simulink model "Casc_Filter_x4"  (Simulink 6.6)
settings: Solver=ode45  StartTime=0.0  StopTime=4100/sampling_freq  RelTol=1e-3
values from neighbouring files (symbols this model uses):
  filter_clk = sampling_freq*clk_mult    (= 144000000)    [Casecade_Taps.m]
  h_g = round(h_g*2^17)/2^17    [Casecade_Taps.m]
  h_k = round(h_k*2^17)/2^17    [Casecade_Taps.m]
  sampling_freq = 48e6    (= 48000000)    [Casecade_Taps.m]
undefined symbols (not defined in the file or in its folder): A, B, Fs, get, PCIN
libraries: xbsIndex_r4 x839, dspsnks4 x5, dspsrcs4 x1, simulink x1
(part 7 of 8)

== system Casc_Filter_x4/DDC/DDC C/Gaussian FIR Filters/Gaussian FIR Filter/Symmetric Data Flow ==
  Data In : Inport
  Counter : Inport  Port=2
  Counter Inv : Inport  Port=3
  Symmetric Shift Register : Subsystem
  Symmetric Shift Register1 : Subsystem
  Symmetric Shift Register2 : Subsystem
  Data 1 : Outport
  Data 2 : Outport  Port=2
  Data 3 : Outport  Port=3
  wires:
  Symmetric Shift Register/1(Shift Out 1) -> Symmetric Shift Register1/1(Shift In 1)
  Symmetric Shift Register1/3(Shift Out 2) -> Symmetric Shift Register/4(Shift In 2)
  Symmetric Shift Register/2(Sum Out) -> Data 1/1
  Symmetric Shift Register1/2(Sum Out) -> Data 2/1
  Data In/1 -> Symmetric Shift Register/1(Shift In 1)
  Counter/1 -> Symmetric Shift Register1/2(Counter), Symmetric Shift Register2/2(Counter), Symmetric Shift Register/2(Counter)
  Symmetric Shift Register1/1(Shift Out 1) -> Symmetric Shift Register2/1(Shift In 1)
  Symmetric Shift Register2/2(Sum Out) -> Data 3/1
  Symmetric Shift Register2/1(Shift Out 1) -> Symmetric Shift Register2/4(Shift In 2)
  Symmetric Shift Register2/3(Shift Out 2) -> Symmetric Shift Register1/4(Shift In 2)
  Counter Inv/1 -> Symmetric Shift Register/3(Counter Inv), Symmetric Shift Register1/3(Counter Inv), Symmetric Shift Register2/3(Counter Inv)

== system Casc_Filter_x4/DDC/DDC C/Gaussian FIR Filters/Gaussian FIR Filter1/Gaussian Accumulate ==
  Counter : Inport
  Data In : Inport  Port=2
  Constant : xbsIndex_r4/Constant  arith_type=Signed (2's comp)  const=0  n_bits=1  bin_pt=0  explicit_period=off  period=1  equ=P=C  opselect=C  inp2=PCIN>>17  opr=+  inp1=P  carry=CIN  dbl_ovrd=off  block_type=constant
      settings: block_version=VER_STRING_GOES_HERE
  Constant1 : xbsIndex_r4/Constant  arith_type=Signed (2's comp)  const=131071  n_bits=48  bin_pt=0  explicit_period=off  period=1  equ=P=P+1  opselect=Custom  inp2=P  opr=+  inp1=0  carry=1  dbl_ovrd=off  block_type=constant
      settings: block_version=VER_STRING_GOES_HERE
  Constant11 : xbsIndex_r4/Constant  arith_type=DSP48 Instruction  const=5  n_bits=7  bin_pt=0  explicit_period=off  period=1  equ=P=PCIN+(P)  opselect=Custom  inp2=PCIN  opr=+  inp1=P  carry=0  dbl_ovrd=off  block_type=constant
      settings: block_version=VER_STRING_GOES_HERE
  Constant2 : xbsIndex_r4/Constant  arith_type=Signed (2's comp)  const=0  n_bits=18  bin_pt=0  explicit_period=off  period=1  equ=P=P+1  opselect=Custom  inp2=P  opr=+  inp1=0  carry=1  dbl_ovrd=off  block_type=constant
      settings: block_version=VER_STRING_GOES_HERE
  Constant3 : xbsIndex_r4/Constant  arith_type=DSP48 Instruction  const=5  n_bits=7  bin_pt=0  explicit_period=off  period=1  equ=P=PCIN+(C)  opselect=Custom  inp2=PCIN  opr=+  inp1=C  carry=0  dbl_ovrd=off  block_type=constant
      settings: block_version=VER_STRING_GOES_HERE
  Constant6 : xbsIndex_r4/Constant  arith_type=Signed (2's comp)  const=0  n_bits=18  bin_pt=0  explicit_period=off  period=1  equ=P=P+1  opselect=Custom  inp2=P  opr=+  inp1=0  carry=1  dbl_ovrd=off  block_type=constant
      settings: block_version=VER_STRING_GOES_HERE
  DSP48 : xbsIndex_r4/DSP48  use_b=Direct from B Port  use_op=on  use_creg=on  use_pcin=on  use_pcout=off  use_bcout=off  rst_all=off  en_all=off  pipeline_a=0  pipeline_b=0  pipeline_c=off  pipeline_p=on  pipeline_mult=off  pipeline_opmode=on  pipeline_sub=off  pipeline_carryin=off  pipeline_carryinsel=off  rst_a=off  rst_b=off  rst_c=off  rst_mult=off  rst_p=off  rst_carry_in=off  rst_ctrl=off  en_a=off  en_b=off  en_c=off  en_mult=off  en_p=off  en_carry_in=off  en_ctrl=off  dbl_ovrd=off  use_synth_model=off  xl_useadderonly=on  block_type=dsp48
      settings: block_version=VER_STRING_GOES_HERE
  Delay1 : xbsIndex_r4/Delay  Orientation=down  en=off  latency=2  dbl_ovrd=off  reg_retiming=off  block_type=delay
      settings: infoedit=Hardware notes: A delay line is a chain, each link of which is an SRL16 followed by a flip-flop. If register retiming is enabled, the delay line is a chain of flip-flops.  block_version=VER_STRING_GOES_HERE
  Down Sample : xbsIndex_r4/Down Sample  sample_ratio=12  sample_phase="Last Value of Frame  (most efficient)"  en=off  latency=1  dbl_ovrd=off  block_type=dsamp
      settings: xl_area=[8 16 0 0 0 0 0]  block_version=VER_STRING_GOES_HERE
  Mux1 : xbsIndex_r4/Mux  inputs=2  en=off  latency=1  precision=Full  arith_type=Unsigned  n_bits=16  bin_pt=14  quantization=Truncate  overflow=Wrap  dbl_ovrd=off  block_type=mux
      settings: xl_area=[63 0 0 126 0 0 0]  block_version=VER_STRING_GOES_HERE
  Register : xbsIndex_r4/Register  Orientation=down  init=0  rst=off  en=on  dbl_ovrd=off  block_type=register
      settings: xl_area=[9 18 0 0 0 0 0]  block_version=VER_STRING_GOES_HERE
  Register1 : xbsIndex_r4/Register  init=0  rst=off  en=off  dbl_ovrd=off  block_type=register
      settings: block_version=8.2
  Reinterpret : xbsIndex_r4/Reinterpret  force_arith_type=on  arith_type="Signed  (2's comp)"  force_bin_pt=on  bin_pt=15  block_type=reinterpret
      settings: infoedit="Changes signal type without altering the binary representation.   You can changed the signal between signed and unsigned, and relocate the binary point.<P><P>Hardware notes: In hardware this block costs nothing.<P><P>Example:  Suppose the input is 6 bits wide, signed, with 2 fractional bits, and the output is forced to unsigned with 0 fractional bits.  Then an input of -2.0 (1110.00 in binary 2's complement) becomes an output of 56 (111000 in binary)."  block_version=8.2
  Relational : xbsIndex_r4/Relational  mode=a=b  en=off  latency=5  dbl_ovrd=off  block_type=relational
      settings: xl_area=[5 2 0 10 0 0 0]  block_version=VER_STRING_GOES_HERE
  Slice : xbsIndex_r4/Slice  nbits=16  boolean_output=off  mode=Lower Bit Location + Width  bit1=0  base1=MSB of Input  bit0=18  base0=LSB of Input  dbl_ovrd=off  block_type=slice
      settings: infoedit="Extracts a given range of bits from each input sample and presents it at the output.  The output type is ordinarily unsigned with binary point at zero, but can be Boolean when the slice is one bit wide.<P><P>Hardware notes: In hardware this block costs nothing."  block_version=VER_STRING_GOES_HERE
  Data Out : Outport
  wires:
  Constant/1 -> Relational/2
  Relational/1 -> Delay1/1, Mux1/1
  Counter/1 -> Relational/1
  Register/1 -> Down Sample/1
  Down Sample/1 -> Slice/1
  Delay1/1 -> Register/2
  Constant2/1 -> DSP48/1
  Constant6/1 -> DSP48/2
  Constant11/1 -> Mux1/2
  Constant3/1 -> Mux1/3
  DSP48/1 -> Register/1
  Slice/1 -> Reinterpret/1
  Register1/1 -> Data Out/1
  Mux1/1 -> DSP48/5
  Data In/1 -> DSP48/4
  Constant1/1 -> DSP48/3
  Reinterpret/1 -> Register1/1

== system Casc_Filter_x4/DDC/DDC C/Gaussian FIR Filters/Gaussian FIR Filter1/Gaussian Mult ==
  Data 1 : Inport
  Data 2 : Inport  Port=2
  Data 3 : Inport  Port=3
  Coeff 1 : Inport  Port=4
  Coeff 2 : Inport  Port=5
  Coeff 3 : Inport  Port=6
  Constant1 : xbsIndex_r4/Constant  arith_type=DSP48 Instruction  const=53  n_bits=7  bin_pt=0  explicit_period=off  period=1  equ=P=PCIN+(A*B)  opselect=PCIN + A*B  inp2=PCIN>>17  opr=+  inp1=P  carry=CIN  dbl_ovrd=off  block_type=constant
      settings: block_version=VER_STRING_GOES_HERE
  Constant2 : xbsIndex_r4/Constant  arith_type=DSP48 Instruction  const=53  n_bits=7  bin_pt=0  explicit_period=off  period=1  equ=P=PCIN+(A*B)  opselect=PCIN + A*B  inp2=PCIN>>17  opr=+  inp1=P  carry=CIN  dbl_ovrd=off  block_type=constant
      settings: block_version=VER_STRING_GOES_HERE
  Constant3 : xbsIndex_r4/Constant  arith_type=DSP48 Instruction  const=5  n_bits=7  bin_pt=0  explicit_period=off  period=1  equ=P=+(A*B)  opselect=A * B  inp2=PCIN>>17  opr=+  inp1=P  carry=CIN  dbl_ovrd=off  block_type=constant
      settings: block_version=VER_STRING_GOES_HERE
  DSP1 : xbsIndex_r4/DSP48  use_b=Direct from B Port  use_op=on  use_creg=off  use_pcin=on  use_pcout=on  use_bcout=off  rst_all=off  en_all=off  pipeline_a=2  pipeline_b=2  pipeline_c=on  pipeline_p=on  pipeline_mult=on  pipeline_opmode=off  pipeline_sub=off  pipeline_carryin=off  pipeline_carryinsel=off  rst_a=off  rst_b=off  rst_c=off  rst_mult=off  rst_p=off  rst_carry_in=off  rst_ctrl=off  en_a=off  en_b=off  en_c=off  en_mult=off  en_p=off  en_carry_in=off  en_ctrl=off  dbl_ovrd=off  use_synth_model=off  xl_useadderonly=off  block_type=dsp48
      settings: block_version=VER_STRING_GOES_HERE
  DSP3 : xbsIndex_r4/DSP48  use_b=Direct from B Port  use_op=on  use_creg=off  use_pcin=off  use_pcout=on  use_bcout=off  rst_all=off  en_all=off  pipeline_a=1  pipeline_b=1  pipeline_c=off  pipeline_p=on  pipeline_mult=on  pipeline_opmode=off  pipeline_sub=off  pipeline_carryin=off  pipeline_carryinsel=off  rst_a=off  rst_b=off  rst_c=off  rst_mult=off  rst_p=off  rst_carry_in=off  rst_ctrl=off  en_a=off  en_b=off  en_c=off  en_mult=off  en_p=off  en_carry_in=off  en_ctrl=off  dbl_ovrd=off  use_synth_model=off  xl_useadderonly=off  block_type=dsp48
      settings: block_version=VER_STRING_GOES_HERE
  DSP48 : xbsIndex_r4/DSP48  use_b=Direct from B Port  use_op=on  use_creg=off  use_pcin=on  use_pcout=on  use_bcout=off  rst_all=off  en_all=off  pipeline_a=2  pipeline_b=2  pipeline_c=on  pipeline_p=on  pipeline_mult=on  pipeline_opmode=off  pipeline_sub=off  pipeline_carryin=off  pipeline_carryinsel=off  rst_a=off  rst_b=off  rst_c=off  rst_mult=off  rst_p=off  rst_carry_in=off  rst_ctrl=off  en_a=off  en_b=off  en_c=off  en_mult=off  en_p=off  en_carry_in=off  en_ctrl=off  dbl_ovrd=off  use_synth_model=off  xl_useadderonly=off  block_type=dsp48
      settings: block_version=VER_STRING_GOES_HERE
  Delay1 : xbsIndex_r4/Delay  en=off  latency=2  dbl_ovrd=off  reg_retiming=off  block_type=delay
      settings: infoedit=Hardware notes: A delay line is a chain, each link of which is an SRL16 followed by a flip-flop. If register retiming is enabled, the delay line is a chain of flip-flops.  xl_area=[9 18 0 18 0 0 0]  block_version=VER_STRING_GOES_HERE
  Delay2 : xbsIndex_r4/Delay  en=off  latency=2  dbl_ovrd=off  reg_retiming=off  block_type=delay
      settings: infoedit=Hardware notes: A delay line is a chain, each link of which is an SRL16 followed by a flip-flop. If register retiming is enabled, the delay line is a chain of flip-flops.  xl_area=[9 18 0 18 0 0 0]  block_version=VER_STRING_GOES_HERE
  Delay3 : xbsIndex_r4/Delay  en=off  latency=3  dbl_ovrd=off  reg_retiming=off  block_type=delay
      settings: infoedit=Hardware notes: A delay line is a chain, each link of which is an SRL16 followed by a flip-flop. If register retiming is enabled, the delay line is a chain of flip-flops.  xl_area=[9 18 0 18 0 0 0]  block_version=VER_STRING_GOES_HERE
  Delay6 : xbsIndex_r4/Delay  en=off  latency=1  dbl_ovrd=off  reg_retiming=off  block_type=delay
      settings: infoedit=Hardware notes: A delay line is a chain, each link of which is an SRL16 followed by a flip-flop. If register retiming is enabled, the delay line is a chain of flip-flops.  xl_area=[9 18 0 18 0 0 0]  block_version=VER_STRING_GOES_HERE
  Reinterpret{,1..5} (6 alike) : xbsIndex_r4/Reinterpret  force_arith_type=on  arith_type="Signed  (2's comp)"  force_bin_pt=on  bin_pt=0  block_type=cast
      settings: infoedit="Changes type of samples without altering their binary representation.<P><P>Hardware notes: In hardware this block costs nothing.<P><P>Example:  Suppose the input is 6 bits wide, signed, with 2 fractional bits, and the output is forced to unsigned with 0 fractional bits.  Then an input of -2.0 (1110.00 in binary 2's complement) becomes an output of 56 (111000 in binary)."  block_version=VER_STRING_GOES_HERE
  Terminator : Terminator
  Terminator1 : Terminator
  Terminator2 : Terminator
  Sum Out : Outport
  wires:
  Data 1/1 -> Delay6/1
  Coeff 1/1 -> Delay3/1
  Data 3/1 -> Reinterpret/1
  Coeff 3/1 -> Delay1/1
  Delay1/1 -> Reinterpret1/1
  Delay3/1 -> Reinterpret5/1
  Delay6/1 -> Reinterpret4/1
  Coeff 2/1 -> Delay2/1
  Data 2/1 -> Reinterpret2/1
  Delay2/1 -> Reinterpret3/1
  Reinterpret/1 -> DSP3/1
  Reinterpret1/1 -> DSP3/2
  Constant3/1 -> DSP3/3
  DSP3/2 -> DSP48/3
  DSP3/1 -> Terminator/1
  Constant1/1 -> DSP48/4
  Reinterpret2/1 -> DSP48/1
  Reinterpret3/1 -> DSP48/2
  DSP48/2 -> DSP1/3
  DSP48/1 -> Terminator1/1
  Constant2/1 -> DSP1/4
  Reinterpret4/1 -> DSP1/1
  Reinterpret5/1 -> DSP1/2
  DSP1/1 -> Terminator2/1
  DSP1/2 -> Sum Out/1

== system Casc_Filter_x4/DDC/DDC C/Gaussian FIR Filters/Gaussian FIR Filter1/Symmetric Data Flow ==
  Data In : Inport
  Counter : Inport  Port=2
  Counter Inv : Inport  Port=3
  Symmetric Shift Register : Subsystem
  Symmetric Shift Register1 : Subsystem
  Symmetric Shift Register2 : Subsystem
  Data 1 : Outport
  Data 2 : Outport  Port=2
  Data 3 : Outport  Port=3
  wires:
  Symmetric Shift Register/1(Shift Out 1) -> Symmetric Shift Register1/1(Shift In 1)
  Symmetric Shift Register1/3(Shift Out 2) -> Symmetric Shift Register/4(Shift In 2)
  Symmetric Shift Register/2(Sum Out) -> Data 1/1
  Symmetric Shift Register1/2(Sum Out) -> Data 2/1
  Data In/1 -> Symmetric Shift Register/1(Shift In 1)
  Counter/1 -> Symmetric Shift Register1/2(Counter), Symmetric Shift Register2/2(Counter), Symmetric Shift Register/2(Counter)
  Symmetric Shift Register1/1(Shift Out 1) -> Symmetric Shift Register2/1(Shift In 1)
  Symmetric Shift Register2/2(Sum Out) -> Data 3/1
  Symmetric Shift Register2/1(Shift Out 1) -> Symmetric Shift Register2/4(Shift In 2)
  Symmetric Shift Register2/3(Shift Out 2) -> Symmetric Shift Register1/4(Shift In 2)
  Counter Inv/1 -> Symmetric Shift Register/3(Counter Inv), Symmetric Shift Register1/3(Counter Inv), Symmetric Shift Register2/3(Counter Inv)

== system Casc_Filter_x4/DDC/DDC A/Gaussian FIR Filters/Gaussian FIR Filter/Symmetric Data Flow/Symmetric Shift Register ==
  Shift In 1 : Inport
  Counter : Inport  Port=2
  Counter Inv : Inport  Port=3
  Shift In 2 : Inport  Port=4
  ASR : xbsIndex_r4/Addressable Shift Register  infer_latency=off  depth=12  initVector=[0]  en=off  dbl_ovrd=off  use_behavioral_HDL=off  use_rpm=off  block_type=addrsr
      settings: infoedit="Delay of  configurable length.  Any element  in the delay     line   can    be   addressed   and   driven    onto   the   output     port.<P><P>Hardware  notes: Implemented  using SRL16s.     If Virtex-4, Virtex-II or Spartan-3 devices are used, multiple SRLC16s are cascaded together."  xl_area=[9 0 0 18 0 0 0]  block_version=VER_STRING_GOES_HERE
  ASR1 : xbsIndex_r4/Addressable Shift Register  infer_latency=off  depth=12  initVector=[0]  en=off  dbl_ovrd=off  use_behavioral_HDL=off  use_rpm=off  block_type=addrsr
      settings: infoedit="Delay of  configurable length.  Any element  in the delay     line   can    be   addressed   and   driven    onto   the   output     port.<P><P>Hardware  notes: Implemented  using SRL16s.     If Virtex-4, Virtex-II or Spartan-3 devices are used, multiple SRLC16s are cascaded together."  xl_area=[9 0 0 18 0 0 0]  block_version=VER_STRING_GOES_HERE
  AddSub : xbsIndex_r4/AddSub  mode=Addition  use_carryin=off  use_carryout=off  en=off  latency=1  precision=User Defined  arith_type="Signed  (2's comp)"  n_bits=18  bin_pt=16  quantization="Round  (unbiased: +/- Inf)"  overflow=Saturate  dbl_ovrd=off  use_behavioral_HDL=off  pipelined=on  use_rpm=on  block_type=addsub
      settings: xl_area=[19 0 0 37 0 0 0]  block_version=VER_STRING_GOES_HERE
  Delay : xbsIndex_r4/Delay  en=off  latency=12  dbl_ovrd=off  reg_retiming=off  block_type=delay
      settings: infoedit=Hardware notes: A delay line is a chain, each link of which is an SRL16 followed by a flip-flop. If register retiming is enabled, the delay line is a chain of flip-flops.  xl_area=[9 18 0 18 0 0 0]  block_version=VER_STRING_GOES_HERE
  Delay1 : xbsIndex_r4/Delay  en=off  latency=12  dbl_ovrd=off  reg_retiming=off  block_type=delay
      settings: infoedit=Hardware notes: A delay line is a chain, each link of which is an SRL16 followed by a flip-flop. If register retiming is enabled, the delay line is a chain of flip-flops.  xl_area=[9 18 0 18 0 0 0]  block_version=VER_STRING_GOES_HERE
  Register : xbsIndex_r4/Register  init=0  rst=off  en=off  dbl_ovrd=off  block_type=register
      settings: block_version=8.2
  Register1 : xbsIndex_r4/Register  init=0  rst=off  en=off  dbl_ovrd=off  block_type=register
      settings: block_version=8.2
  Shift Out 1 : Outport
  Sum Out : Outport  Port=2
  Shift Out 2 : Outport  Port=3
  wires:
  Counter Inv/1 -> ASR1/2
  Shift In 1/1 -> ASR/1, Delay/1
  Shift In 2/1 -> Delay1/1, ASR1/1
  Counter/1 -> ASR/2
  ASR/1 -> Register/1
  ASR1/1 -> Register1/1
  AddSub/1 -> Sum Out/1
  Delay1/1 -> Shift Out 2/1
  Delay/1 -> Shift Out 1/1
  Register/1 -> AddSub/1
  Register1/1 -> AddSub/2

== system Casc_Filter_x4/DDC/DDC A/Gaussian FIR Filters/Gaussian FIR Filter/Symmetric Data Flow/Symmetric Shift Register1 ==
  Shift In 1 : Inport
  Counter : Inport  Port=2
  Counter Inv : Inport  Port=3
  Shift In 2 : Inport  Port=4
  ASR : xbsIndex_r4/Addressable Shift Register  infer_latency=off  depth=12  initVector=[0]  en=off  dbl_ovrd=off  use_behavioral_HDL=off  use_rpm=off  block_type=addrsr
      settings: infoedit="Delay of  configurable length.  Any element  in the delay     line   can    be   addressed   and   driven    onto   the   output     port.<P><P>Hardware  notes: Implemented  using SRL16s.     If Virtex-4, Virtex-II or Spartan-3 devices are used, multiple SRLC16s are cascaded together."  xl_area=[9 0 0 18 0 0 0]  block_version=VER_STRING_GOES_HERE
  ASR1 : xbsIndex_r4/Addressable Shift Register  infer_latency=off  depth=12  initVector=[0]  en=off  dbl_ovrd=off  use_behavioral_HDL=off  use_rpm=off  block_type=addrsr
      settings: infoedit="Delay of  configurable length.  Any element  in the delay     line   can    be   addressed   and   driven    onto   the   output     port.<P><P>Hardware  notes: Implemented  using SRL16s.     If Virtex-4, Virtex-II or Spartan-3 devices are used, multiple SRLC16s are cascaded together."  xl_area=[9 0 0 18 0 0 0]  block_version=VER_STRING_GOES_HERE
  AddSub : xbsIndex_r4/AddSub  mode=Addition  use_carryin=off  use_carryout=off  en=off  latency=1  precision=User Defined  arith_type="Signed  (2's comp)"  n_bits=18  bin_pt=16  quantization="Round  (unbiased: +/- Inf)"  overflow=Saturate  dbl_ovrd=off  use_behavioral_HDL=off  pipelined=on  use_rpm=on  block_type=addsub
      settings: xl_area=[19 0 0 37 0 0 0]  block_version=VER_STRING_GOES_HERE
  Delay : xbsIndex_r4/Delay  en=off  latency=12  dbl_ovrd=off  reg_retiming=off  block_type=delay
      settings: infoedit=Hardware notes: A delay line is a chain, each link of which is an SRL16 followed by a flip-flop. If register retiming is enabled, the delay line is a chain of flip-flops.  xl_area=[9 18 0 18 0 0 0]  block_version=VER_STRING_GOES_HERE
  Delay1 : xbsIndex_r4/Delay  en=off  latency=12  dbl_ovrd=off  reg_retiming=off  block_type=delay
      settings: infoedit=Hardware notes: A delay line is a chain, each link of which is an SRL16 followed by a flip-flop. If register retiming is enabled, the delay line is a chain of flip-flops.  xl_area=[9 18 0 18 0 0 0]  block_version=VER_STRING_GOES_HERE
  Register : xbsIndex_r4/Register  init=0  rst=off  en=off  dbl_ovrd=off  block_type=register
      settings: block_version=8.2
  Register1 : xbsIndex_r4/Register  init=0  rst=off  en=off  dbl_ovrd=off  block_type=register
      settings: block_version=8.2
  Shift Out 1 : Outport
  Sum Out : Outport  Port=2
  Shift Out 2 : Outport  Port=3
  wires:
  Counter Inv/1 -> ASR1/2
  Shift In 1/1 -> ASR/1, Delay/1
  Shift In 2/1 -> Delay1/1, ASR1/1
  Counter/1 -> ASR/2
  ASR/1 -> Register/1
  ASR1/1 -> Register1/1
  AddSub/1 -> Sum Out/1
  Delay1/1 -> Shift Out 2/1
  Delay/1 -> Shift Out 1/1
  Register/1 -> AddSub/1
  Register1/1 -> AddSub/2

== system Casc_Filter_x4/DDC/DDC A/Gaussian FIR Filters/Gaussian FIR Filter/Symmetric Data Flow/Symmetric Shift Register2 ==
  Shift In 1 : Inport
  Counter : Inport  Port=2
  Counter Inv : Inport  Port=3
  Shift In 2 : Inport  Port=4
  ASR : xbsIndex_r4/Addressable Shift Register  infer_latency=off  depth=12  initVector=[0]  en=off  dbl_ovrd=off  use_behavioral_HDL=off  use_rpm=off  block_type=addrsr
      settings: infoedit="Delay of  configurable length.  Any element  in the delay     line   can    be   addressed   and   driven    onto   the   output     port.<P><P>Hardware  notes: Implemented  using SRL16s.     If Virtex-4, Virtex-II or Spartan-3 devices are used, multiple SRLC16s are cascaded together."  xl_area=[9 0 0 18 0 0 0]  block_version=VER_STRING_GOES_HERE
  ASR1 : xbsIndex_r4/Addressable Shift Register  infer_latency=off  depth=12  initVector=[0]  en=off  dbl_ovrd=off  use_behavioral_HDL=off  use_rpm=off  block_type=addrsr
      settings: infoedit="Delay of  configurable length.  Any element  in the delay     line   can    be   addressed   and   driven    onto   the   output     port.<P><P>Hardware  notes: Implemented  using SRL16s.     If Virtex-4, Virtex-II or Spartan-3 devices are used, multiple SRLC16s are cascaded together."  xl_area=[9 0 0 18 0 0 0]  block_version=VER_STRING_GOES_HERE
  AddSub : xbsIndex_r4/AddSub  mode=Addition  use_carryin=off  use_carryout=off  en=off  latency=1  precision=User Defined  arith_type="Signed  (2's comp)"  n_bits=18  bin_pt=16  quantization="Round  (unbiased: +/- Inf)"  overflow=Saturate  dbl_ovrd=off  use_behavioral_HDL=off  pipelined=on  use_rpm=on  block_type=addsub
      settings: xl_area=[19 0 0 37 0 0 0]  block_version=VER_STRING_GOES_HERE
  Delay : xbsIndex_r4/Delay  en=off  latency=12  dbl_ovrd=off  reg_retiming=off  block_type=delay
      settings: infoedit=Hardware notes: A delay line is a chain, each link of which is an SRL16 followed by a flip-flop. If register retiming is enabled, the delay line is a chain of flip-flops.  xl_area=[9 18 0 18 0 0 0]  block_version=VER_STRING_GOES_HERE
  Delay1 : xbsIndex_r4/Delay  en=off  latency=12  dbl_ovrd=off  reg_retiming=off  block_type=delay
      settings: infoedit=Hardware notes: A delay line is a chain, each link of which is an SRL16 followed by a flip-flop. If register retiming is enabled, the delay line is a chain of flip-flops.  xl_area=[9 18 0 18 0 0 0]  block_version=VER_STRING_GOES_HERE
  Register : xbsIndex_r4/Register  init=0  rst=off  en=off  dbl_ovrd=off  block_type=register
      settings: block_version=8.2
  Register1 : xbsIndex_r4/Register  init=0  rst=off  en=off  dbl_ovrd=off  block_type=register
      settings: block_version=8.2
  Shift Out 1 : Outport
  Sum Out : Outport  Port=2
  Shift Out 2 : Outport  Port=3
  wires:
  Counter Inv/1 -> ASR1/2
  Shift In 1/1 -> ASR/1, Delay/1
  Shift In 2/1 -> Delay1/1, ASR1/1
  Counter/1 -> ASR/2
  ASR/1 -> Register/1
  ASR1/1 -> Register1/1
  AddSub/1 -> Sum Out/1
  Delay1/1 -> Shift Out 2/1
  Delay/1 -> Shift Out 1/1
  Register/1 -> AddSub/1
  Register1/1 -> AddSub/2

== system Casc_Filter_x4/DDC/DDC A/Gaussian FIR Filters/Gaussian FIR Filter1/Symmetric Data Flow/Symmetric Shift Register ==
  Shift In 1 : Inport
  Counter : Inport  Port=2
  Counter Inv : Inport  Port=3
  Shift In 2 : Inport  Port=4
  ASR : xbsIndex_r4/Addressable Shift Register  infer_latency=off  depth=12  initVector=[0]  en=off  dbl_ovrd=off  use_behavioral_HDL=off  use_rpm=off  block_type=addrsr
      settings: infoedit="Delay of  configurable length.  Any element  in the delay     line   can    be   addressed   and   driven    onto   the   output     port.<P><P>Hardware  notes: Implemented  using SRL16s.     If Virtex-4, Virtex-II or Spartan-3 devices are used, multiple SRLC16s are cascaded together."  xl_area=[9 0 0 18 0 0 0]  block_version=VER_STRING_GOES_HERE
  ASR1 : xbsIndex_r4/Addressable Shift Register  infer_latency=off  depth=12  initVector=[0]  en=off  dbl_ovrd=off  use_behavioral_HDL=off  use_rpm=off  block_type=addrsr
      settings: infoedit="Delay of  configurable length.  Any element  in the delay     line   can    be   addressed   and   driven    onto   the   output     port.<P><P>Hardware  notes: Implemented  using SRL16s.     If Virtex-4, Virtex-II or Spartan-3 devices are used, multiple SRLC16s are cascaded together."  xl_area=[9 0 0 18 0 0 0]  block_version=VER_STRING_GOES_HERE
  AddSub : xbsIndex_r4/AddSub  mode=Addition  use_carryin=off  use_carryout=off  en=off  latency=1  precision=User Defined  arith_type="Signed  (2's comp)"  n_bits=18  bin_pt=16  quantization="Round  (unbiased: +/- Inf)"  overflow=Saturate  dbl_ovrd=off  use_behavioral_HDL=off  pipelined=on  use_rpm=on  block_type=addsub
      settings: xl_area=[19 0 0 37 0 0 0]  block_version=VER_STRING_GOES_HERE
  Delay : xbsIndex_r4/Delay  en=off  latency=12  dbl_ovrd=off  reg_retiming=off  block_type=delay
      settings: infoedit=Hardware notes: A delay line is a chain, each link of which is an SRL16 followed by a flip-flop. If register retiming is enabled, the delay line is a chain of flip-flops.  xl_area=[9 18 0 18 0 0 0]  block_version=VER_STRING_GOES_HERE
  Delay1 : xbsIndex_r4/Delay  en=off  latency=12  dbl_ovrd=off  reg_retiming=off  block_type=delay
      settings: infoedit=Hardware notes: A delay line is a chain, each link of which is an SRL16 followed by a flip-flop. If register retiming is enabled, the delay line is a chain of flip-flops.  xl_area=[9 18 0 18 0 0 0]  block_version=VER_STRING_GOES_HERE
  Register : xbsIndex_r4/Register  init=0  rst=off  en=off  dbl_ovrd=off  block_type=register
      settings: block_version=8.2
  Register1 : xbsIndex_r4/Register  init=0  rst=off  en=off  dbl_ovrd=off  block_type=register
      settings: block_version=8.2
  Shift Out 1 : Outport
  Sum Out : Outport  Port=2
  Shift Out 2 : Outport  Port=3
  wires:
  Counter Inv/1 -> ASR1/2
  Shift In 1/1 -> ASR/1, Delay/1
  Shift In 2/1 -> Delay1/1, ASR1/1
  Counter/1 -> ASR/2
  ASR/1 -> Register/1
  ASR1/1 -> Register1/1
  AddSub/1 -> Sum Out/1
  Delay1/1 -> Shift Out 2/1
  Delay/1 -> Shift Out 1/1
  Register/1 -> AddSub/1
  Register1/1 -> AddSub/2

== system Casc_Filter_x4/DDC/DDC A/Gaussian FIR Filters/Gaussian FIR Filter1/Symmetric Data Flow/Symmetric Shift Register1 ==
  Shift In 1 : Inport
  Counter : Inport  Port=2
  Counter Inv : Inport  Port=3
  Shift In 2 : Inport  Port=4
  ASR : xbsIndex_r4/Addressable Shift Register  infer_latency=off  depth=12  initVector=[0]  en=off  dbl_ovrd=off  use_behavioral_HDL=off  use_rpm=off  block_type=addrsr
      settings: infoedit="Delay of  configurable length.  Any element  in the delay     line   can    be   addressed   and   driven    onto   the   output     port.<P><P>Hardware  notes: Implemented  using SRL16s.     If Virtex-4, Virtex-II or Spartan-3 devices are used, multiple SRLC16s are cascaded together."  xl_area=[9 0 0 18 0 0 0]  block_version=VER_STRING_GOES_HERE
  ASR1 : xbsIndex_r4/Addressable Shift Register  infer_latency=off  depth=12  initVector=[0]  en=off  dbl_ovrd=off  use_behavioral_HDL=off  use_rpm=off  block_type=addrsr
      settings: infoedit="Delay of  configurable length.  Any element  in the delay     line   can    be   addressed   and   driven    onto   the   output     port.<P><P>Hardware  notes: Implemented  using SRL16s.     If Virtex-4, Virtex-II or Spartan-3 devices are used, multiple SRLC16s are cascaded together."  xl_area=[9 0 0 18 0 0 0]  block_version=VER_STRING_GOES_HERE
  AddSub : xbsIndex_r4/AddSub  mode=Addition  use_carryin=off  use_carryout=off  en=off  latency=1  precision=User Defined  arith_type="Signed  (2's comp)"  n_bits=18  bin_pt=16  quantization="Round  (unbiased: +/- Inf)"  overflow=Saturate  dbl_ovrd=off  use_behavioral_HDL=off  pipelined=on  use_rpm=on  block_type=addsub
      settings: xl_area=[19 0 0 37 0 0 0]  block_version=VER_STRING_GOES_HERE
  Delay : xbsIndex_r4/Delay  en=off  latency=12  dbl_ovrd=off  reg_retiming=off  block_type=delay
      settings: infoedit=Hardware notes: A delay line is a chain, each link of which is an SRL16 followed by a flip-flop. If register retiming is enabled, the delay line is a chain of flip-flops.  xl_area=[9 18 0 18 0 0 0]  block_version=VER_STRING_GOES_HERE
  Delay1 : xbsIndex_r4/Delay  en=off  latency=12  dbl_ovrd=off  reg_retiming=off  block_type=delay
      settings: infoedit=Hardware notes: A delay line is a chain, each link of which is an SRL16 followed by a flip-flop. If register retiming is enabled, the delay line is a chain of flip-flops.  xl_area=[9 18 0 18 0 0 0]  block_version=VER_STRING_GOES_HERE
  Register : xbsIndex_r4/Register  init=0  rst=off  en=off  dbl_ovrd=off  block_type=register
      settings: block_version=8.2
  Register1 : xbsIndex_r4/Register  init=0  rst=off  en=off  dbl_ovrd=off  block_type=register
      settings: block_version=8.2
  Shift Out 1 : Outport
  Sum Out : Outport  Port=2
  Shift Out 2 : Outport  Port=3
  wires:
  Counter Inv/1 -> ASR1/2
  Shift In 1/1 -> ASR/1, Delay/1
  Shift In 2/1 -> Delay1/1, ASR1/1
  Counter/1 -> ASR/2
  ASR/1 -> Register/1
  ASR1/1 -> Register1/1
  AddSub/1 -> Sum Out/1
  Delay1/1 -> Shift Out 2/1
  Delay/1 -> Shift Out 1/1
  Register/1 -> AddSub/1
  Register1/1 -> AddSub/2

== system Casc_Filter_x4/DDC/DDC A/Gaussian FIR Filters/Gaussian FIR Filter1/Symmetric Data Flow/Symmetric Shift Register2 ==
  Shift In 1 : Inport
  Counter : Inport  Port=2
  Counter Inv : Inport  Port=3
  Shift In 2 : Inport  Port=4
  ASR : xbsIndex_r4/Addressable Shift Register  infer_latency=off  depth=12  initVector=[0]  en=off  dbl_ovrd=off  use_behavioral_HDL=off  use_rpm=off  block_type=addrsr
      settings: infoedit="Delay of  configurable length.  Any element  in the delay     line   can    be   addressed   and   driven    onto   the   output     port.<P><P>Hardware  notes: Implemented  using SRL16s.     If Virtex-4, Virtex-II or Spartan-3 devices are used, multiple SRLC16s are cascaded together."  xl_area=[9 0 0 18 0 0 0]  block_version=VER_STRING_GOES_HERE
  ASR1 : xbsIndex_r4/Addressable Shift Register  infer_latency=off  depth=12  initVector=[0]  en=off  dbl_ovrd=off  use_behavioral_HDL=off  use_rpm=off  block_type=addrsr
      settings: infoedit="Delay of  configurable length.  Any element  in the delay     line   can    be   addressed   and   driven    onto   the   output     port.<P><P>Hardware  notes: Implemented  using SRL16s.     If Virtex-4, Virtex-II or Spartan-3 devices are used, multiple SRLC16s are cascaded together."  xl_area=[9 0 0 18 0 0 0]  block_version=VER_STRING_GOES_HERE
  AddSub : xbsIndex_r4/AddSub  mode=Addition  use_carryin=off  use_carryout=off  en=off  latency=1  precision=User Defined  arith_type="Signed  (2's comp)"  n_bits=18  bin_pt=16  quantization="Round  (unbiased: +/- Inf)"  overflow=Saturate  dbl_ovrd=off  use_behavioral_HDL=off  pipelined=on  use_rpm=on  block_type=addsub
      settings: xl_area=[19 0 0 37 0 0 0]  block_version=VER_STRING_GOES_HERE
  Delay : xbsIndex_r4/Delay  en=off  latency=12  dbl_ovrd=off  reg_retiming=off  block_type=delay
      settings: infoedit=Hardware notes: A delay line is a chain, each link of which is an SRL16 followed by a flip-flop. If register retiming is enabled, the delay line is a chain of flip-flops.  xl_area=[9 18 0 18 0 0 0]  block_version=VER_STRING_GOES_HERE
  Delay1 : xbsIndex_r4/Delay  en=off  latency=12  dbl_ovrd=off  reg_retiming=off  block_type=delay
      settings: infoedit=Hardware notes: A delay line is a chain, each link of which is an SRL16 followed by a flip-flop. If register retiming is enabled, the delay line is a chain of flip-flops.  xl_area=[9 18 0 18 0 0 0]  block_version=VER_STRING_GOES_HERE
  Register : xbsIndex_r4/Register  init=0  rst=off  en=off  dbl_ovrd=off  block_type=register
      settings: block_version=8.2
  Register1 : xbsIndex_r4/Register  init=0  rst=off  en=off  dbl_ovrd=off  block_type=register
      settings: block_version=8.2
  Shift Out 1 : Outport
  Sum Out : Outport  Port=2
  Shift Out 2 : Outport  Port=3
  wires:
  Counter Inv/1 -> ASR1/2
  Shift In 1/1 -> ASR/1, Delay/1
  Shift In 2/1 -> Delay1/1, ASR1/1
  Counter/1 -> ASR/2
  ASR/1 -> Register/1
  ASR1/1 -> Register1/1
  AddSub/1 -> Sum Out/1
  Delay1/1 -> Shift Out 2/1
  Delay/1 -> Shift Out 1/1
  Register/1 -> AddSub/1
  Register1/1 -> AddSub/2

== system Casc_Filter_x4/DDC/DDC A1/Gaussian FIR Filters/Gaussian FIR Filter/Symmetric Data Flow/Symmetric Shift Register ==
  Shift In 1 : Inport
  Counter : Inport  Port=2
  Counter Inv : Inport  Port=3
  Shift In 2 : Inport  Port=4
  ASR : xbsIndex_r4/Addressable Shift Register  infer_latency=off  depth=12  initVector=[0]  en=off  dbl_ovrd=off  use_behavioral_HDL=off  use_rpm=off  block_type=addrsr
      settings: infoedit="Delay of  configurable length.  Any element  in the delay     line   can    be   addressed   and   driven    onto   the   output     port.<P><P>Hardware  notes: Implemented  using SRL16s.     If Virtex-4, Virtex-II or Spartan-3 devices are used, multiple SRLC16s are cascaded together."  xl_area=[9 0 0 18 0 0 0]  block_version=VER_STRING_GOES_HERE
  ASR1 : xbsIndex_r4/Addressable Shift Register  infer_latency=off  depth=12  initVector=[0]  en=off  dbl_ovrd=off  use_behavioral_HDL=off  use_rpm=off  block_type=addrsr
      settings: infoedit="Delay of  configurable length.  Any element  in the delay     line   can    be   addressed   and   driven    onto   the   output     port.<P><P>Hardware  notes: Implemented  using SRL16s.     If Virtex-4, Virtex-II or Spartan-3 devices are used, multiple SRLC16s are cascaded together."  xl_area=[9 0 0 18 0 0 0]  block_version=VER_STRING_GOES_HERE
  AddSub : xbsIndex_r4/AddSub  mode=Addition  use_carryin=off  use_carryout=off  en=off  latency=1  precision=User Defined  arith_type="Signed  (2's comp)"  n_bits=18  bin_pt=16  quantization="Round  (unbiased: +/- Inf)"  overflow=Saturate  dbl_ovrd=off  use_behavioral_HDL=off  pipelined=on  use_rpm=on  block_type=addsub
      settings: xl_area=[19 0 0 37 0 0 0]  block_version=VER_STRING_GOES_HERE
  Delay : xbsIndex_r4/Delay  en=off  latency=12  dbl_ovrd=off  reg_retiming=off  block_type=delay
      settings: infoedit=Hardware notes: A delay line is a chain, each link of which is an SRL16 followed by a flip-flop. If register retiming is enabled, the delay line is a chain of flip-flops.  xl_area=[9 18 0 18 0 0 0]  block_version=VER_STRING_GOES_HERE
  Delay1 : xbsIndex_r4/Delay  en=off  latency=12  dbl_ovrd=off  reg_retiming=off  block_type=delay
      settings: infoedit=Hardware notes: A delay line is a chain, each link of which is an SRL16 followed by a flip-flop. If register retiming is enabled, the delay line is a chain of flip-flops.  xl_area=[9 18 0 18 0 0 0]  block_version=VER_STRING_GOES_HERE
  Register : xbsIndex_r4/Register  init=0  rst=off  en=off  dbl_ovrd=off  block_type=register
      settings: block_version=8.2
  Register1 : xbsIndex_r4/Register  init=0  rst=off  en=off  dbl_ovrd=off  block_type=register
      settings: block_version=8.2
  Shift Out 1 : Outport
  Sum Out : Outport  Port=2
  Shift Out 2 : Outport  Port=3
  wires:
  Counter Inv/1 -> ASR1/2
  Shift In 1/1 -> ASR/1, Delay/1
  Shift In 2/1 -> Delay1/1, ASR1/1
  Counter/1 -> ASR/2
  ASR/1 -> Register/1
  ASR1/1 -> Register1/1
  AddSub/1 -> Sum Out/1
  Delay1/1 -> Shift Out 2/1
  Delay/1 -> Shift Out 1/1
  Register/1 -> AddSub/1
  Register1/1 -> AddSub/2

== system Casc_Filter_x4/DDC/DDC A1/Gaussian FIR Filters/Gaussian FIR Filter/Symmetric Data Flow/Symmetric Shift Register1 ==
  Shift In 1 : Inport
  Counter : Inport  Port=2
  Counter Inv : Inport  Port=3
  Shift In 2 : Inport  Port=4
  ASR : xbsIndex_r4/Addressable Shift Register  infer_latency=off  depth=12  initVector=[0]  en=off  dbl_ovrd=off  use_behavioral_HDL=off  use_rpm=off  block_type=addrsr
      settings: infoedit="Delay of  configurable length.  Any element  in the delay     line   can    be   addressed   and   driven    onto   the   output     port.<P><P>Hardware  notes: Implemented  using SRL16s.     If Virtex-4, Virtex-II or Spartan-3 devices are used, multiple SRLC16s are cascaded together."  xl_area=[9 0 0 18 0 0 0]  block_version=VER_STRING_GOES_HERE
  ASR1 : xbsIndex_r4/Addressable Shift Register  infer_latency=off  depth=12  initVector=[0]  en=off  dbl_ovrd=off  use_behavioral_HDL=off  use_rpm=off  block_type=addrsr
      settings: infoedit="Delay of  configurable length.  Any element  in the delay     line   can    be   addressed   and   driven    onto   the   output     port.<P><P>Hardware  notes: Implemented  using SRL16s.     If Virtex-4, Virtex-II or Spartan-3 devices are used, multiple SRLC16s are cascaded together."  xl_area=[9 0 0 18 0 0 0]  block_version=VER_STRING_GOES_HERE
  AddSub : xbsIndex_r4/AddSub  mode=Addition  use_carryin=off  use_carryout=off  en=off  latency=1  precision=User Defined  arith_type="Signed  (2's comp)"  n_bits=18  bin_pt=16  quantization="Round  (unbiased: +/- Inf)"  overflow=Saturate  dbl_ovrd=off  use_behavioral_HDL=off  pipelined=on  use_rpm=on  block_type=addsub
      settings: xl_area=[19 0 0 37 0 0 0]  block_version=VER_STRING_GOES_HERE
  Delay : xbsIndex_r4/Delay  en=off  latency=12  dbl_ovrd=off  reg_retiming=off  block_type=delay
      settings: infoedit=Hardware notes: A delay line is a chain, each link of which is an SRL16 followed by a flip-flop. If register retiming is enabled, the delay line is a chain of flip-flops.  xl_area=[9 18 0 18 0 0 0]  block_version=VER_STRING_GOES_HERE
  Delay1 : xbsIndex_r4/Delay  en=off  latency=12  dbl_ovrd=off  reg_retiming=off  block_type=delay
      settings: infoedit=Hardware notes: A delay line is a chain, each link of which is an SRL16 followed by a flip-flop. If register retiming is enabled, the delay line is a chain of flip-flops.  xl_area=[9 18 0 18 0 0 0]  block_version=VER_STRING_GOES_HERE
  Register : xbsIndex_r4/Register  init=0  rst=off  en=off  dbl_ovrd=off  block_type=register
      settings: block_version=8.2
  Register1 : xbsIndex_r4/Register  init=0  rst=off  en=off  dbl_ovrd=off  block_type=register
      settings: block_version=8.2
  Shift Out 1 : Outport
  Sum Out : Outport  Port=2
  Shift Out 2 : Outport  Port=3
  wires:
  Counter Inv/1 -> ASR1/2
  Shift In 1/1 -> ASR/1, Delay/1
  Shift In 2/1 -> Delay1/1, ASR1/1
  Counter/1 -> ASR/2
  ASR/1 -> Register/1
  ASR1/1 -> Register1/1
  AddSub/1 -> Sum Out/1
  Delay1/1 -> Shift Out 2/1
  Delay/1 -> Shift Out 1/1
  Register/1 -> AddSub/1
  Register1/1 -> AddSub/2

== system Casc_Filter_x4/DDC/DDC A1/Gaussian FIR Filters/Gaussian FIR Filter/Symmetric Data Flow/Symmetric Shift Register2 ==
  Shift In 1 : Inport
  Counter : Inport  Port=2
  Counter Inv : Inport  Port=3
  Shift In 2 : Inport  Port=4
  ASR : xbsIndex_r4/Addressable Shift Register  infer_latency=off  depth=12  initVector=[0]  en=off  dbl_ovrd=off  use_behavioral_HDL=off  use_rpm=off  block_type=addrsr
      settings: infoedit="Delay of  configurable length.  Any element  in the delay     line   can    be   addressed   and   driven    onto   the   output     port.<P><P>Hardware  notes: Implemented  using SRL16s.     If Virtex-4, Virtex-II or Spartan-3 devices are used, multiple SRLC16s are cascaded together."  xl_area=[9 0 0 18 0 0 0]  block_version=VER_STRING_GOES_HERE
  ASR1 : xbsIndex_r4/Addressable Shift Register  infer_latency=off  depth=12  initVector=[0]  en=off  dbl_ovrd=off  use_behavioral_HDL=off  use_rpm=off  block_type=addrsr
      settings: infoedit="Delay of  configurable length.  Any element  in the delay     line   can    be   addressed   and   driven    onto   the   output     port.<P><P>Hardware  notes: Implemented  using SRL16s.     If Virtex-4, Virtex-II or Spartan-3 devices are used, multiple SRLC16s are cascaded together."  xl_area=[9 0 0 18 0 0 0]  block_version=VER_STRING_GOES_HERE
  AddSub : xbsIndex_r4/AddSub  mode=Addition  use_carryin=off  use_carryout=off  en=off  latency=1  precision=User Defined  arith_type="Signed  (2's comp)"  n_bits=18  bin_pt=16  quantization="Round  (unbiased: +/- Inf)"  overflow=Saturate  dbl_ovrd=off  use_behavioral_HDL=off  pipelined=on  use_rpm=on  block_type=addsub
      settings: xl_area=[19 0 0 37 0 0 0]  block_version=VER_STRING_GOES_HERE
  Delay : xbsIndex_r4/Delay  en=off  latency=12  dbl_ovrd=off  reg_retiming=off  block_type=delay
      settings: infoedit=Hardware notes: A delay line is a chain, each link of which is an SRL16 followed by a flip-flop. If register retiming is enabled, the delay line is a chain of flip-flops.  xl_area=[9 18 0 18 0 0 0]  block_version=VER_STRING_GOES_HERE
  Delay1 : xbsIndex_r4/Delay  en=off  latency=12  dbl_ovrd=off  reg_retiming=off  block_type=delay
      settings: infoedit=Hardware notes: A delay line is a chain, each link of which is an SRL16 followed by a flip-flop. If register retiming is enabled, the delay line is a chain of flip-flops.  xl_area=[9 18 0 18 0 0 0]  block_version=VER_STRING_GOES_HERE
  Register : xbsIndex_r4/Register  init=0  rst=off  en=off  dbl_ovrd=off  block_type=register
      settings: block_version=8.2
  Register1 : xbsIndex_r4/Register  init=0  rst=off  en=off  dbl_ovrd=off  block_type=register
      settings: block_version=8.2
  Shift Out 1 : Outport
  Sum Out : Outport  Port=2
  Shift Out 2 : Outport  Port=3
  wires:
  Counter Inv/1 -> ASR1/2
  Shift In 1/1 -> ASR/1, Delay/1
  Shift In 2/1 -> Delay1/1, ASR1/1
  Counter/1 -> ASR/2
  ASR/1 -> Register/1
  ASR1/1 -> Register1/1
  AddSub/1 -> Sum Out/1
  Delay1/1 -> Shift Out 2/1
  Delay/1 -> Shift Out 1/1
  Register/1 -> AddSub/1
  Register1/1 -> AddSub/2

== system Casc_Filter_x4/DDC/DDC A1/Gaussian FIR Filters/Gaussian FIR Filter1/Symmetric Data Flow/Symmetric Shift Register ==
  Shift In 1 : Inport
  Counter : Inport  Port=2
  Counter Inv : Inport  Port=3
  Shift In 2 : Inport  Port=4
  ASR : xbsIndex_r4/Addressable Shift Register  infer_latency=off  depth=12  initVector=[0]  en=off  dbl_ovrd=off  use_behavioral_HDL=off  use_rpm=off  block_type=addrsr
      settings: infoedit="Delay of  configurable length.  Any element  in the delay     line   can    be   addressed   and   driven    onto   the   output     port.<P><P>Hardware  notes: Implemented  using SRL16s.     If Virtex-4, Virtex-II or Spartan-3 devices are used, multiple SRLC16s are cascaded together."  xl_area=[9 0 0 18 0 0 0]  block_version=VER_STRING_GOES_HERE
  ASR1 : xbsIndex_r4/Addressable Shift Register  infer_latency=off  depth=12  initVector=[0]  en=off  dbl_ovrd=off  use_behavioral_HDL=off  use_rpm=off  block_type=addrsr
      settings: infoedit="Delay of  configurable length.  Any element  in the delay     line   can    be   addressed   and   driven    onto   the   output     port.<P><P>Hardware  notes: Implemented  using SRL16s.     If Virtex-4, Virtex-II or Spartan-3 devices are used, multiple SRLC16s are cascaded together."  xl_area=[9 0 0 18 0 0 0]  block_version=VER_STRING_GOES_HERE
  AddSub : xbsIndex_r4/AddSub  mode=Addition  use_carryin=off  use_carryout=off  en=off  latency=1  precision=User Defined  arith_type="Signed  (2's comp)"  n_bits=18  bin_pt=16  quantization="Round  (unbiased: +/- Inf)"  overflow=Saturate  dbl_ovrd=off  use_behavioral_HDL=off  pipelined=on  use_rpm=on  block_type=addsub
      settings: xl_area=[19 0 0 37 0 0 0]  block_version=VER_STRING_GOES_HERE
  Delay : xbsIndex_r4/Delay  en=off  latency=12  dbl_ovrd=off  reg_retiming=off  block_type=delay
      settings: infoedit=Hardware notes: A delay line is a chain, each link of which is an SRL16 followed by a flip-flop. If register retiming is enabled, the delay line is a chain of flip-flops.  xl_area=[9 18 0 18 0 0 0]  block_version=VER_STRING_GOES_HERE
  Delay1 : xbsIndex_r4/Delay  en=off  latency=12  dbl_ovrd=off  reg_retiming=off  block_type=delay
      settings: infoedit=Hardware notes: A delay line is a chain, each link of which is an SRL16 followed by a flip-flop. If register retiming is enabled, the delay line is a chain of flip-flops.  xl_area=[9 18 0 18 0 0 0]  block_version=VER_STRING_GOES_HERE
  Register : xbsIndex_r4/Register  init=0  rst=off  en=off  dbl_ovrd=off  block_type=register
      settings: block_version=8.2
  Register1 : xbsIndex_r4/Register  init=0  rst=off  en=off  dbl_ovrd=off  block_type=register
      settings: block_version=8.2
  Shift Out 1 : Outport
  Sum Out : Outport  Port=2
  Shift Out 2 : Outport  Port=3
  wires:
  Counter Inv/1 -> ASR1/2
  Shift In 1/1 -> ASR/1, Delay/1
  Shift In 2/1 -> Delay1/1, ASR1/1
  Counter/1 -> ASR/2
  ASR/1 -> Register/1
  ASR1/1 -> Register1/1
  AddSub/1 -> Sum Out/1
  Delay1/1 -> Shift Out 2/1
  Delay/1 -> Shift Out 1/1
  Register/1 -> AddSub/1
  Register1/1 -> AddSub/2

== system Casc_Filter_x4/DDC/DDC A1/Gaussian FIR Filters/Gaussian FIR Filter1/Symmetric Data Flow/Symmetric Shift Register1 ==
  Shift In 1 : Inport
  Counter : Inport  Port=2
  Counter Inv : Inport  Port=3
  Shift In 2 : Inport  Port=4
  ASR : xbsIndex_r4/Addressable Shift Register  infer_latency=off  depth=12  initVector=[0]  en=off  dbl_ovrd=off  use_behavioral_HDL=off  use_rpm=off  block_type=addrsr
      settings: infoedit="Delay of  configurable length.  Any element  in the delay     line   can    be   addressed   and   driven    onto   the   output     port.<P><P>Hardware  notes: Implemented  using SRL16s.     If Virtex-4, Virtex-II or Spartan-3 devices are used, multiple SRLC16s are cascaded together."  xl_area=[9 0 0 18 0 0 0]  block_version=VER_STRING_GOES_HERE
  ASR1 : xbsIndex_r4/Addressable Shift Register  infer_latency=off  depth=12  initVector=[0]  en=off  dbl_ovrd=off  use_behavioral_HDL=off  use_rpm=off  block_type=addrsr
      settings: infoedit="Delay of  configurable length.  Any element  in the delay     line   can    be   addressed   and   driven    onto   the   output     port.<P><P>Hardware  notes: Implemented  using SRL16s.     If Virtex-4, Virtex-II or Spartan-3 devices are used, multiple SRLC16s are cascaded together."  xl_area=[9 0 0 18 0 0 0]  block_version=VER_STRING_GOES_HERE
  AddSub : xbsIndex_r4/AddSub  mode=Addition  use_carryin=off  use_carryout=off  en=off  latency=1  precision=User Defined  arith_type="Signed  (2's comp)"  n_bits=18  bin_pt=16  quantization="Round  (unbiased: +/- Inf)"  overflow=Saturate  dbl_ovrd=off  use_behavioral_HDL=off  pipelined=on  use_rpm=on  block_type=addsub
      settings: xl_area=[19 0 0 37 0 0 0]  block_version=VER_STRING_GOES_HERE
  Delay : xbsIndex_r4/Delay  en=off  latency=12  dbl_ovrd=off  reg_retiming=off  block_type=delay
      settings: infoedit=Hardware notes: A delay line is a chain, each link of which is an SRL16 followed by a flip-flop. If register retiming is enabled, the delay line is a chain of flip-flops.  xl_area=[9 18 0 18 0 0 0]  block_version=VER_STRING_GOES_HERE
  Delay1 : xbsIndex_r4/Delay  en=off  latency=12  dbl_ovrd=off  reg_retiming=off  block_type=delay
      settings: infoedit=Hardware notes: A delay line is a chain, each link of which is an SRL16 followed by a flip-flop. If register retiming is enabled, the delay line is a chain of flip-flops.  xl_area=[9 18 0 18 0 0 0]  block_version=VER_STRING_GOES_HERE
  Register : xbsIndex_r4/Register  init=0  rst=off  en=off  dbl_ovrd=off  block_type=register
      settings: block_version=8.2
  Register1 : xbsIndex_r4/Register  init=0  rst=off  en=off  dbl_ovrd=off  block_type=register
      settings: block_version=8.2
  Shift Out 1 : Outport
  Sum Out : Outport  Port=2
  Shift Out 2 : Outport  Port=3
  wires:
  Counter Inv/1 -> ASR1/2
  Shift In 1/1 -> ASR/1, Delay/1
  Shift In 2/1 -> Delay1/1, ASR1/1
  Counter/1 -> ASR/2
  ASR/1 -> Register/1
  ASR1/1 -> Register1/1
  AddSub/1 -> Sum Out/1
  Delay1/1 -> Shift Out 2/1
  Delay/1 -> Shift Out 1/1
  Register/1 -> AddSub/1
  Register1/1 -> AddSub/2
